simulink model "main"  (R2018b)
settings: Solver=VariableStepAuto  StartTime=0.0  StopTime=200  RelTol=1e-3
libraries: simulink x6, aerolibutil x2, sharedtransform x2
settings Model: SimulationMode=accelerator  Creator=exote  LastModifiedBy=exote

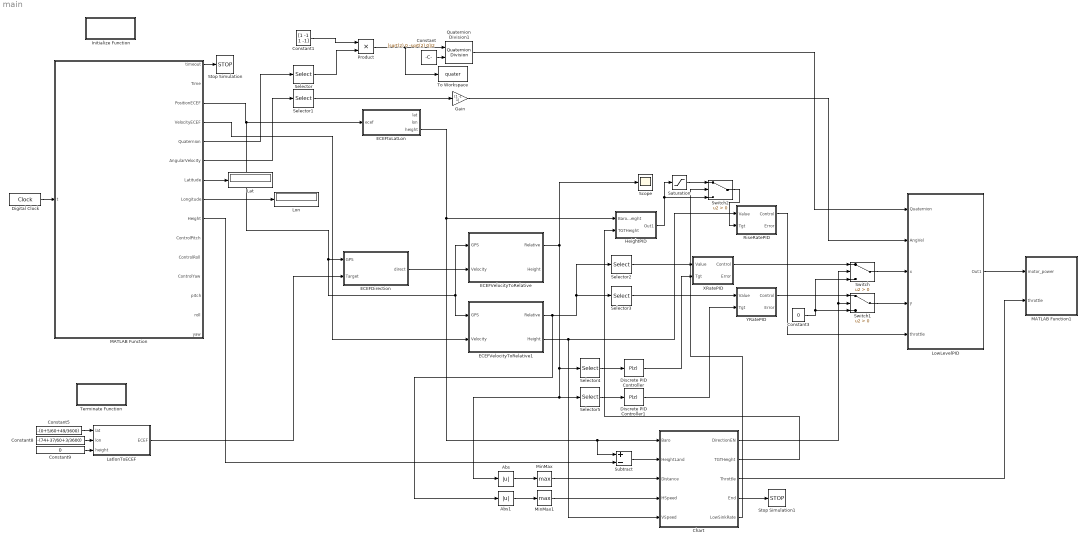
== system main ==
  Abs : Abs
  Abs1 : Abs
  Chart : Stateflow chart  TreatAsAtomicUnit=on
  Constant : Constant  Value=[sqrt(2) 0 -sqrt(2) 0]/2
  Constant1 : Constant  Value=[1 -1 1 -1]
  Constant3 : Constant  Value=0
  Constant5 : Constant  Value=-(0+5/60+49/3600)
  Constant8 : Constant  Value=-(74+37/60+3/3600)
  Constant9 : Constant  Value=0
  Digital Clock : DigitalClock  SampleTime=0.01
  Discrete PID Controller : simulink/Continuous/PID Controller  Controller=P  Form=Parallel  TimeDomain=Discrete-time  SampleTime=-1  IntegratorMethod=Forward Euler  FilterMethod=Forward Euler  ControllerParametersSource=internal  P=-0.1  I=0  D=0  UseFilter=on  N=100  TunerSelectOption=Transfer Function Based (PID Tuner App)  InitialConditionSource=internal  InitialConditionForIntegrator=0  InitialConditionForFilter=0  DifferentiatorICPrevScaledInput=0  ExternalReset=none  TrackingMode=off  Kt=1  LimitOutput=on  UpperSaturationLimit=20  LowerSaturationLimit=-20  LinearizeAsGain=off  AntiWindupMode=none  Kb=1  POutMin=[]  POutMax=[]  IOutMin=[]  IOutMax=[]  DOutMin=[]  DOutMax=[]  NOutMin=[]  NOutMax=[]  SumOutMin=[]  SumOutMax=[]  SaturationOutMin=[]  SaturationOutMax=[]  PParamMin=[]  PParamMax=[]  IParamMin=[]  IParamMax=[]  DParamMin=[]  DParamMax=[]  NParamMin=[]  NParamMax=[]  KbParamMin=[]  KbParamMax=[]  KtParamMin=[]  KtParamMax=[]  KbOutMin=[]  KbOutMax=[]  KtOutMin=[]  KtOutMax=[]  IntegratorOutMin=[]  IntegratorOutMax=[]  FilterOutMin=[]  FilterOutMax=[]  SumI1OutMin=[]  SumI1OutMax=[]  SumI2OutMin=[]  SumI2OutMax=[]  SumI3OutMin=[]  SumI3OutMax=[]  SumI4OutMin=[]  SumI4OutMax=[]  SumDOutMin=[]  SumDOutMax=[]  DifferentiatorOutMin=[]  DifferentiatorOutMax=[]  FilterDiffOutCoefMin=[]  FilterDiffOutCoefMax=[]  ReciprocalOutMin=[]  ReciprocalOutMax=[]  SumDenOutMin=[]  SumDenOutMax=[]  SumNumOutMin=[]  SumNumOutMax=[]  DivideOutMin=[]  DivideOutMax=[]  IntegratorContinuousStateAttributes=''  IntegratorStateMustResolveToSignalObject=off  IntegratorRTWStateStorageClass=Auto  FilterContinuousStateAttributes=''  FilterStateMustResolveToSignalObject=off  FilterRTWStateStorageClass=Auto  ParallelPVariant=InternalParameters  IdealPVariant=Disabled  IVariant=Disabled  DVariant=Disabled  IntegratorVariant=Disabled  SatVariant=Enabled  AWVariant=Disabled  PCopyVariant=Disabled  TRVariant=Disabled  FdbkBlocksVariant=Forward  IdealPFdbkVariant=Disabled  SatFdbkVariant=Disabled  DerivativeFilterVariant=Disabled  NVariant=Disabled  NCopyVariant=Disabled_SignalSpec  FilterICVariant=Disabled  IntegratorICVariant=Disabled  ExternalResetVariant=Disabled  TRSumVariant=Passthrough  SumFdbkVariant=Disabled  SumVariant=Passthrough_P
  Discrete PID Controller1 : simulink/Continuous/PID Controller  Controller=P  Form=Parallel  TimeDomain=Discrete-time  SampleTime=-1  IntegratorMethod=Forward Euler  FilterMethod=Forward Euler  ControllerParametersSource=internal  P=-0.1  I=0  D=0  UseFilter=on  N=100  TunerSelectOption=Transfer Function Based (PID Tuner App)  InitialConditionSource=internal  InitialConditionForIntegrator=0  InitialConditionForFilter=0  DifferentiatorICPrevScaledInput=0  ExternalReset=none  TrackingMode=off  Kt=1  LimitOutput=on  UpperSaturationLimit=20  LowerSaturationLimit=-20  LinearizeAsGain=off  AntiWindupMode=none  Kb=1  POutMin=[]  POutMax=[]  IOutMin=[]  IOutMax=[]  DOutMin=[]  DOutMax=[]  NOutMin=[]  NOutMax=[]  SumOutMin=[]  SumOutMax=[]  SaturationOutMin=[]  SaturationOutMax=[]  PParamMin=[]  PParamMax=[]  IParamMin=[]  IParamMax=[]  DParamMin=[]  DParamMax=[]  NParamMin=[]  NParamMax=[]  KbParamMin=[]  KbParamMax=[]  KtParamMin=[]  KtParamMax=[]  KbOutMin=[]  KbOutMax=[]  KtOutMin=[]  KtOutMax=[]  IntegratorOutMin=[]  IntegratorOutMax=[]  FilterOutMin=[]  FilterOutMax=[]  SumI1OutMin=[]  SumI1OutMax=[]  SumI2OutMin=[]  SumI2OutMax=[]  SumI3OutMin=[]  SumI3OutMax=[]  SumI4OutMin=[]  SumI4OutMax=[]  SumDOutMin=[]  SumDOutMax=[]  DifferentiatorOutMin=[]  DifferentiatorOutMax=[]  FilterDiffOutCoefMin=[]  FilterDiffOutCoefMax=[]  ReciprocalOutMin=[]  ReciprocalOutMax=[]  SumDenOutMin=[]  SumDenOutMax=[]  SumNumOutMin=[]  SumNumOutMax=[]  DivideOutMin=[]  DivideOutMax=[]  IntegratorContinuousStateAttributes=''  IntegratorStateMustResolveToSignalObject=off  IntegratorRTWStateStorageClass=Auto  FilterContinuousStateAttributes=''  FilterStateMustResolveToSignalObject=off  FilterRTWStateStorageClass=Auto  ParallelPVariant=InternalParameters  IdealPVariant=Disabled  IVariant=Disabled  DVariant=Disabled  IntegratorVariant=Disabled  SatVariant=Enabled  AWVariant=Disabled  PCopyVariant=Disabled  TRVariant=Disabled  FdbkBlocksVariant=Forward  IdealPFdbkVariant=Disabled  SatFdbkVariant=Disabled  DerivativeFilterVariant=Disabled  NVariant=Disabled  NCopyVariant=Disabled_SignalSpec  FilterICVariant=Disabled  IntegratorICVariant=Disabled  ExternalResetVariant=Disabled  TRSumVariant=Passthrough  SumFdbkVariant=Disabled  SumVariant=Passthrough_P
  ECEFDirection : MATLAB Function  TreatAsAtomicUnit=on
  ECEFVelocityToRelative : MATLAB Function  TreatAsAtomicUnit=on
  ECEFVelocityToRelative1 : MATLAB Function  TreatAsAtomicUnit=on
  ECEFtoLatLon : MATLAB Function  TreatAsAtomicUnit=on
  Gain : Gain  Gain=[1 -1 1]
  HeightPID : Subsystem
  Initialize Function : Subsystem  TreatAsAtomicUnit=on
  Lat : Display
  "LatlonToECEF " : MATLAB Function  TreatAsAtomicUnit=on
  Lon : Display
  "LowLevelPID " : Subsystem
  MATLAB Function : MATLAB Function  TreatAsAtomicUnit=on
  MATLAB Function1 : MATLAB Function  TreatAsAtomicUnit=on
  MinMax : MinMax  Function=max
  MinMax1 : MinMax  Function=max
  Product : Product
  Quaternion Division1 : aerolibutil/Quaternion Division
      settings: SourceProductName=Aerospace Blockset  SourceProductBaseCode=AE
  "RiseRatePID " : Subsystem
  Saturation : Saturate  UpperLimit=inf
  Scope : Scope
  Selector : Selector  InputPortWidth=4  IndexOptions=Index vector (dialog)  Indices=[4 1 2 3]  OutputSizes=1
  Selector1 : Selector  InputPortWidth=3  IndexOptions=Index vector (dialog)  Indices=[1 3 2]  OutputSizes=1
  Selector2 : Selector  InputPortWidth=2  IndexOptions=Index vector (dialog)  Indices=1  OutputSizes=1
  Selector3 : Selector  InputPortWidth=2  IndexOptions=Index vector (dialog)  Indices=2  OutputSizes=1
  Selector4 : Selector  InputPortWidth=2  IndexOptions=Index vector (dialog)  Indices=1  OutputSizes=1
  Selector5 : Selector  InputPortWidth=2  IndexOptions=Index vector (dialog)  Indices=2  OutputSizes=1
  Stop Simulation : Stop
  Stop Simulation1 : Stop
  Subtract : Sum  Inputs=+-
  Switch : Switch  Criteria=u2 > Threshold
  Switch1 : Switch  Criteria=u2 > Threshold
  Switch2 : Switch  Criteria=u2 > Threshold
  Terminate Function : Subsystem  TreatAsAtomicUnit=on
  To Workspace : ToWorkspace  VariableName=quater  SampleTime=-1
      settings: Save2DSignal=2-D array (concatenate along first dimension)
  XRatePID : Subsystem
  YRatePID : Subsystem
  wires:
  Digital Clock/1 -> MATLAB Function/1(t)
  MATLAB Function/1(timeout) -> Stop Simulation/1
  Selector/1 -> Product/2
  Constant/1 -> Quaternion Division1/2
  MATLAB Function/5(Quaternion) -> Selector/1
  MATLAB Function/6(AngularVelocity) -> Selector1/1
  Constant1/1 -> Product/1
  Product/1 -> Quaternion Division1/1, To Workspace/1
  Quaternion Division1/1 -> "LowLevelPID "/1("Quaternion ")
  "LowLevelPID "/1(Out1) -> MATLAB Function1/1(motor_power)
  MATLAB Function/7(Latitude) -> Lat/1
  MATLAB Function/8(Longitude) -> Lon/1
  Gain/1 -> "LowLevelPID "/2(AngVel)
  Selector1/1 -> Gain/1
  MATLAB Function/3(PositionECEF) -> ECEFtoLatLon/1(ecef), ECEFVelocityToRelative/1(GPS), ECEFVelocityToRelative1/1(GPS), ECEFDirection/1(GPS)
  MATLAB Function/4(VelocityECEF) -> ECEFVelocityToRelative1/2(Velocity)
  "RiseRatePID "/1(Control) -> "LowLevelPID "/5(throttle)
  ECEFtoLatLon/3(height) -> Chart/1(Baro), Subtract/1, HeightPID/1(BaroHeight)
  Chart/2(TGTHeight) -> HeightPID/2(TGTHeight)
  Constant5/1 -> "LatlonToECEF "/1(lat)
  Constant8/1 -> "LatlonToECEF "/2(lon)
  Constant9/1 -> "LatlonToECEF "/3(height)
  "LatlonToECEF "/1(ECEF) -> ECEFDirection/2(Target)
  ECEFDirection/1(direct) -> ECEFVelocityToRelative/2(Velocity)
  ECEFVelocityToRelative1/2(Height) -> "RiseRatePID "/1("Value "), Chart/5(VSpeed)
  Selector2/1 -> XRatePID/1("Value ")
  Selector3/1 -> YRatePID/1("Value ")
  ECEFVelocityToRelative1/1(Relative) -> Abs1/1, Selector3/1, Selector2/1
  HeightPID/1(Out1) -> Switch2/3, Saturation/1
  YRatePID/1(Control) -> Switch1/1
  XRatePID/1(Control) -> Switch/1
  Selector4/1 -> Discrete PID Controller/1
  Selector5/1 -> Discrete PID Controller1/1
  ECEFVelocityToRelative/1(Relative) -> Abs/1, Selector5/1, Selector4/1, Scope/1
  Discrete PID Controller/1 -> XRatePID/2(Tgt)
  Discrete PID Controller1/1 -> YRatePID/2(Tgt)
  Switch1/1 -> "LowLevelPID "/4(y)
  Switch/1 -> "LowLevelPID "/3(x)
  Constant3/1 -> Switch1/3, Switch/3
  Chart/1(DirectionEN) -> Switch1/2, Switch/2
  Chart/3(Throttle) -> MATLAB Function1/2(throttle)
  MATLAB Function/9(Height) -> Subtract/2
  MinMax/1 -> Chart/3(Distance)
  MinMax1/1 -> Chart/4(HSpeed)
  Chart/4(End) -> Stop Simulation1/1
  Subtract/1 -> Chart/2(HeightLand)
  Abs/1 -> MinMax/1
  Abs1/1 -> MinMax1/1
  Switch2/1 -> "RiseRatePID "/2(Tgt)
  Saturation/1 -> Switch2/1
  Chart/5(LowSinkRate) -> Switch2/2

== system main/HeightPID ==
  BaroHeight : Inport
  TGTHeight : Inport  Port=2
  Discrete PID Controller : simulink/Continuous/PID Controller  Controller=PI  Form=Parallel  TimeDomain=Discrete-time  SampleTime=-1  IntegratorMethod=Forward Euler  FilterMethod=Forward Euler  ControllerParametersSource=internal  P=0.5  I=0  D=0  UseFilter=off  N=100  TunerSelectOption=Transfer Function Based (PID Tuner App)  InitialConditionSource=internal  InitialConditionForIntegrator=0  InitialConditionForFilter=0  DifferentiatorICPrevScaledInput=0  ExternalReset=none  TrackingMode=off  Kt=1  LimitOutput=on  UpperSaturationLimit=20  LowerSaturationLimit=-20  LinearizeAsGain=off  AntiWindupMode=none  Kb=1  POutMin=[]  POutMax=[]  IOutMin=[]  IOutMax=[]  DOutMin=[]  DOutMax=[]  NOutMin=[]  NOutMax=[]  SumOutMin=[]  SumOutMax=[]  SaturationOutMin=[]  SaturationOutMax=[]  PParamMin=[]  PParamMax=[]  IParamMin=[]  IParamMax=[]  DParamMin=[]  DParamMax=[]  NParamMin=[]  NParamMax=[]  KbParamMin=[]  KbParamMax=[]  KtParamMin=[]  KtParamMax=[]  KbOutMin=[]  KbOutMax=[]  KtOutMin=[]  KtOutMax=[]  IntegratorOutMin=[]  IntegratorOutMax=[]  FilterOutMin=[]  FilterOutMax=[]  SumI1OutMin=[]  SumI1OutMax=[]  SumI2OutMin=[]  SumI2OutMax=[]  SumI3OutMin=[]  SumI3OutMax=[]  SumI4OutMin=[]  SumI4OutMax=[]  SumDOutMin=[]  SumDOutMax=[]  DifferentiatorOutMin=[]  DifferentiatorOutMax=[]  FilterDiffOutCoefMin=[]  FilterDiffOutCoefMax=[]  ReciprocalOutMin=[]  ReciprocalOutMax=[]  SumDenOutMin=[]  SumDenOutMax=[]  SumNumOutMin=[]  SumNumOutMax=[]  DivideOutMin=[]  DivideOutMax=[]  IntegratorContinuousStateAttributes=''  IntegratorStateMustResolveToSignalObject=off  IntegratorRTWStateStorageClass=Auto  FilterContinuousStateAttributes=''  FilterStateMustResolveToSignalObject=off  FilterRTWStateStorageClass=Auto  ParallelPVariant=InternalParameters  IdealPVariant=Disabled  IVariant=InternalParameters  DVariant=Disabled  IntegratorVariant=Discrete  SatVariant=Enabled  AWVariant=Passthrough  PCopyVariant=Disabled  TRVariant=Disabled  FdbkBlocksVariant=Forward  IdealPFdbkVariant=Disabled  SatFdbkVariant=Disabled  DerivativeFilterVariant=Disabled  NVariant=Disabled  NCopyVariant=Disabled_SignalSpec  FilterICVariant=Disabled  IntegratorICVariant=InternalICs  ExternalResetVariant=Disabled  TRSumVariant=Passthrough  SumFdbkVariant=Disabled  SumVariant=Sum_PI
  Subtract2 : Sum  Inputs=+-
  Out1 : Outport
  wires:
  Subtract2/1 -> Discrete PID Controller/1
  BaroHeight/1 -> Subtract2/2
  Discrete PID Controller/1 -> Out1/1
  TGTHeight/1 -> Subtract2/1

== system main/Initialize Function ==
  Event Listener : EventListener  DisableCoverage=on  EventName=reset
  MATLAB Function : MATLAB Function  TreatAsAtomicUnit=on

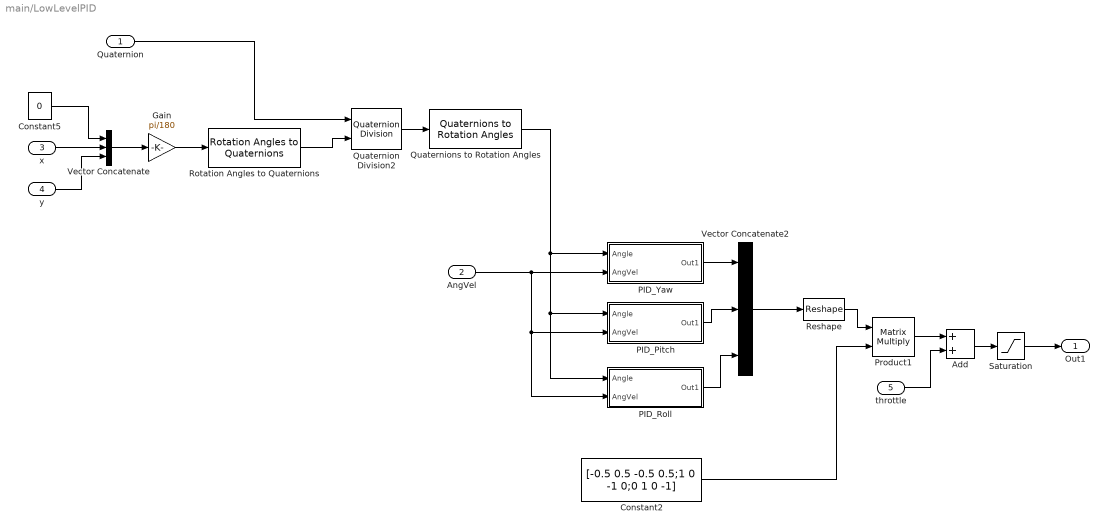
== system main/LowLevelPID  ==
  "Quaternion " : Inport
  AngVel : Inport  Port=2
  x : Inport  Port=3
  y : Inport  Port=4
  throttle : Inport  Port=5
  Add : Sum
  Constant2 : Constant  Value=[-0.5 0.5 -0.5 0.5;1 0 -1 0;0 1 0 -1]
  Constant5 : Constant  Value=0
  Gain : Gain  Gain=pi/180
  PID_Pitch : Subsystem
  PID_Roll : Subsystem
  PID_Yaw : Subsystem
  Product1 : Product  Multiplication=Matrix(*)
  Quaternion Division2 : aerolibutil/Quaternion Division
      settings: SourceProductName=Aerospace Blockset  SourceProductBaseCode=AE
  Quaternions to Rotation Angles : sharedtransform/Quaternions to Rotation Angles  rotationOrder=ZXY  aMode=aMode
      settings: SourceProductBaseCode=AE
  Reshape : Reshape  OutputDimensionality=Customize  OutputDimensions=[1,3]
  Rotation Angles to Quaternions : sharedtransform/Rotation Angles to Quaternions  rotationOrder=ZXY  aMode=aMode
      settings: SourceProductName=Aerospace Blockset  SourceProductBaseCode=AE
  Saturation : Saturate  UpperLimit=1  LowerLimit=0
  Vector Concatenate : Concatenate  NumInputs=3
  Vector Concatenate2 : Concatenate  NumInputs=3
  Out1 : Outport
  wires:
  Product1/1 -> Add/1
  Quaternions to Rotation Angles/1 -> PID_Pitch/1(Angle), PID_Roll/1(Angle), PID_Yaw/1(Angle)
  Vector Concatenate2/1 -> Reshape/1
  Constant2/1 -> Product1/2
  Reshape/1 -> Product1/1
  Add/1 -> Saturation/1
  "Quaternion "/1 -> Quaternion Division2/1
  Rotation Angles to Quaternions/1 -> Quaternion Division2/2
  Quaternion Division2/1 -> Quaternions to Rotation Angles/1
  Saturation/1 -> Out1/1
  throttle/1 -> Add/2
  Vector Concatenate/1 -> Gain/1
  x/1 -> Vector Concatenate/2
  y/1 -> Vector Concatenate/3
  Constant5/1 -> Vector Concatenate/1
  Gain/1 -> Rotation Angles to Quaternions/1
  AngVel/1 -> PID_Roll/2(AngVel), PID_Pitch/2(AngVel), PID_Yaw/2(AngVel)
  PID_Yaw/1(Out1) -> Vector Concatenate2/1
  PID_Pitch/1(Out1) -> Vector Concatenate2/2
  PID_Roll/1(Out1) -> Vector Concatenate2/3

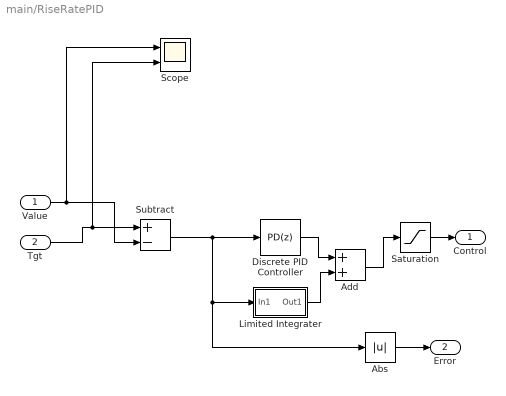
== system main/RiseRatePID  ==
  "Value " : Inport
  Tgt : Inport  Port=2
  Abs : Abs
  Add : Sum
  Discrete PID Controller : simulink/Continuous/PID Controller  Controller=PD  Form=Parallel  TimeDomain=Discrete-time  SampleTime=-1  IntegratorMethod=Forward Euler  FilterMethod=Forward Euler  ControllerParametersSource=internal  P=1  I=1  D=0.01  UseFilter=on  N=30  TunerSelectOption=Transfer Function Based (PID Tuner App)  InitialConditionSource=internal  InitialConditionForIntegrator=0  InitialConditionForFilter=0  DifferentiatorICPrevScaledInput=0  ExternalReset=none  TrackingMode=off  Kt=1  LimitOutput=off  UpperSaturationLimit=0.75  LowerSaturationLimit=0.25  LinearizeAsGain=off  AntiWindupMode=none  Kb=1  POutMin=[]  POutMax=[]  IOutMin=[-100]  IOutMax=[100]  DOutMin=[]  DOutMax=[]  NOutMin=[]  NOutMax=[]  SumOutMin=[]  SumOutMax=[]  SaturationOutMin=[]  SaturationOutMax=[]  PParamMin=[]  PParamMax=[]  IParamMin=[]  IParamMax=[]  DParamMin=[]  DParamMax=[]  NParamMin=[]  NParamMax=[]  KbParamMin=[]  KbParamMax=[]  KtParamMin=[]  KtParamMax=[]  KbOutMin=[]  KbOutMax=[]  KtOutMin=[]  KtOutMax=[]  IntegratorOutMin=[]  IntegratorOutMax=[]  FilterOutMin=[]  FilterOutMax=[]  SumI1OutMin=[]  SumI1OutMax=[]  SumI2OutMin=[]  SumI2OutMax=[]  SumI3OutMin=[]  SumI3OutMax=[]  SumI4OutMin=[]  SumI4OutMax=[]  SumDOutMin=[]  SumDOutMax=[]  DifferentiatorOutMin=[]  DifferentiatorOutMax=[]  FilterDiffOutCoefMin=[]  FilterDiffOutCoefMax=[]  ReciprocalOutMin=[]  ReciprocalOutMax=[]  SumDenOutMin=[]  SumDenOutMax=[]  SumNumOutMin=[]  SumNumOutMax=[]  DivideOutMin=[]  DivideOutMax=[]  IntegratorContinuousStateAttributes=''  IntegratorStateMustResolveToSignalObject=off  IntegratorRTWStateStorageClass=Auto  FilterContinuousStateAttributes=''  FilterStateMustResolveToSignalObject=off  FilterRTWStateStorageClass=Auto  ParallelPVariant=InternalParameters  IdealPVariant=Disabled  IVariant=Disabled  DVariant=InternalParameters  IntegratorVariant=Disabled  SatVariant=Disabled  AWVariant=Disabled  PCopyVariant=Disabled  TRVariant=Disabled  FdbkBlocksVariant=Forward  IdealPFdbkVariant=Disabled  SatFdbkVariant=Disabled  DerivativeFilterVariant=ForwardEulerFilter  NVariant=InternalParameters  NCopyVariant=Disabled  FilterICVariant=InternalICsFilter  IntegratorICVariant=Disabled  ExternalResetVariant=Disabled  TRSumVariant=Passthrough  SumFdbkVariant=Disabled  SumVariant=Sum_PD
  Limited Integrater : Subsystem
  Saturation : Saturate  UpperLimit=0.75  LowerLimit=0.25
  Scope : Scope  NumInputPorts=2
  Subtract : Sum  Inputs=+-
  Control : Outport
  Error : Outport  Port=2
  wires:
  Subtract/1 -> Discrete PID Controller/1, Abs/1, Limited Integrater/1(In1)
  Tgt/1 -> Scope/2, Subtract/1
  Saturation/1 -> Control/1
  Discrete PID Controller/1 -> Add/1
  Limited Integrater/1(Out1) -> Add/2
  Add/1 -> Saturation/1
  "Value "/1 -> Scope/1, Subtract/2
  Abs/1 -> Error/1

== system main/Terminate Function ==
  Event Listener : EventListener  DisableCoverage=on  EventType=Terminate  EventName=reset
  MATLAB Function : MATLAB Function  TreatAsAtomicUnit=on

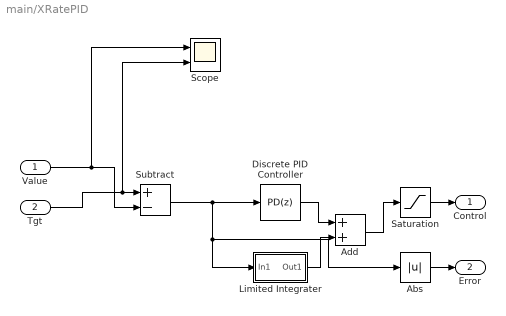
== system main/XRatePID ==
  "Value " : Inport
  Tgt : Inport  Port=2
  Abs : Abs
  Add : Sum
  Discrete PID Controller : simulink/Continuous/PID Controller  Controller=PD  Form=Parallel  TimeDomain=Discrete-time  SampleTime=-1  IntegratorMethod=Forward Euler  FilterMethod=Forward Euler  ControllerParametersSource=internal  P=-5  I=1  D=0  UseFilter=on  N=30  TunerSelectOption=Transfer Function Based (PID Tuner App)  InitialConditionSource=internal  InitialConditionForIntegrator=0  InitialConditionForFilter=0  DifferentiatorICPrevScaledInput=0  ExternalReset=none  TrackingMode=off  Kt=1  LimitOutput=off  UpperSaturationLimit=0.75  LowerSaturationLimit=0.25  LinearizeAsGain=off  AntiWindupMode=none  Kb=1  POutMin=[]  POutMax=[]  IOutMin=[-100]  IOutMax=[100]  DOutMin=[]  DOutMax=[]  NOutMin=[]  NOutMax=[]  SumOutMin=[]  SumOutMax=[]  SaturationOutMin=[]  SaturationOutMax=[]  PParamMin=[]  PParamMax=[]  IParamMin=[]  IParamMax=[]  DParamMin=[]  DParamMax=[]  NParamMin=[]  NParamMax=[]  KbParamMin=[]  KbParamMax=[]  KtParamMin=[]  KtParamMax=[]  KbOutMin=[]  KbOutMax=[]  KtOutMin=[]  KtOutMax=[]  IntegratorOutMin=[]  IntegratorOutMax=[]  FilterOutMin=[]  FilterOutMax=[]  SumI1OutMin=[]  SumI1OutMax=[]  SumI2OutMin=[]  SumI2OutMax=[]  SumI3OutMin=[]  SumI3OutMax=[]  SumI4OutMin=[]  SumI4OutMax=[]  SumDOutMin=[]  SumDOutMax=[]  DifferentiatorOutMin=[]  DifferentiatorOutMax=[]  FilterDiffOutCoefMin=[]  FilterDiffOutCoefMax=[]  ReciprocalOutMin=[]  ReciprocalOutMax=[]  SumDenOutMin=[]  SumDenOutMax=[]  SumNumOutMin=[]  SumNumOutMax=[]  DivideOutMin=[]  DivideOutMax=[]  IntegratorContinuousStateAttributes=''  IntegratorStateMustResolveToSignalObject=off  IntegratorRTWStateStorageClass=Auto  FilterContinuousStateAttributes=''  FilterStateMustResolveToSignalObject=off  FilterRTWStateStorageClass=Auto  ParallelPVariant=InternalParameters  IdealPVariant=Disabled  IVariant=Disabled  DVariant=InternalParameters  IntegratorVariant=Disabled  SatVariant=Disabled  AWVariant=Disabled  PCopyVariant=Disabled  TRVariant=Disabled  FdbkBlocksVariant=Forward  IdealPFdbkVariant=Disabled  SatFdbkVariant=Disabled  DerivativeFilterVariant=ForwardEulerFilter  NVariant=InternalParameters  NCopyVariant=Disabled  FilterICVariant=InternalICsFilter  IntegratorICVariant=Disabled  ExternalResetVariant=Disabled  TRSumVariant=Passthrough  SumFdbkVariant=Disabled  SumVariant=Sum_PD
  Limited Integrater : Subsystem
  Saturation : Saturate  UpperLimit=10  LowerLimit=-10
  Scope : Scope  NumInputPorts=2
  Subtract : Sum  Inputs=+-
  Control : Outport
  Error : Outport  Port=2
  wires:
  Subtract/1 -> Discrete PID Controller/1, Abs/1, Limited Integrater/1(In1)
  Tgt/1 -> Scope/2, Subtract/1
  Saturation/1 -> Control/1
  Discrete PID Controller/1 -> Add/1
  Limited Integrater/1(Out1) -> Add/2
  Add/1 -> Saturation/1
  "Value "/1 -> Scope/1, Subtract/2
  Abs/1 -> Error/1

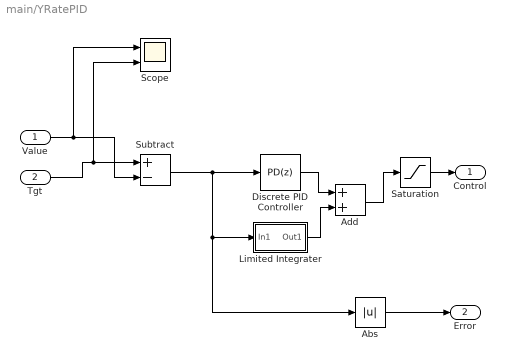
== system main/YRatePID ==
  "Value " : Inport
  Tgt : Inport  Port=2
  Abs : Abs
  Add : Sum
  Discrete PID Controller : simulink/Continuous/PID Controller  Controller=PD  Form=Parallel  TimeDomain=Discrete-time  SampleTime=-1  IntegratorMethod=Forward Euler  FilterMethod=Forward Euler  ControllerParametersSource=internal  P=-5  I=1  D=0  UseFilter=on  N=30  TunerSelectOption=Transfer Function Based (PID Tuner App)  InitialConditionSource=internal  InitialConditionForIntegrator=0  InitialConditionForFilter=0  DifferentiatorICPrevScaledInput=0  ExternalReset=none  TrackingMode=off  Kt=1  LimitOutput=off  UpperSaturationLimit=0.75  LowerSaturationLimit=0.25  LinearizeAsGain=off  AntiWindupMode=none  Kb=1  POutMin=[]  POutMax=[]  IOutMin=[-100]  IOutMax=[100]  DOutMin=[]  DOutMax=[]  NOutMin=[]  NOutMax=[]  SumOutMin=[]  SumOutMax=[]  SaturationOutMin=[]  SaturationOutMax=[]  PParamMin=[]  PParamMax=[]  IParamMin=[]  IParamMax=[]  DParamMin=[]  DParamMax=[]  NParamMin=[]  NParamMax=[]  KbParamMin=[]  KbParamMax=[]  KtParamMin=[]  KtParamMax=[]  KbOutMin=[]  KbOutMax=[]  KtOutMin=[]  KtOutMax=[]  IntegratorOutMin=[]  IntegratorOutMax=[]  FilterOutMin=[]  FilterOutMax=[]  SumI1OutMin=[]  SumI1OutMax=[]  SumI2OutMin=[]  SumI2OutMax=[]  SumI3OutMin=[]  SumI3OutMax=[]  SumI4OutMin=[]  SumI4OutMax=[]  SumDOutMin=[]  SumDOutMax=[]  DifferentiatorOutMin=[]  DifferentiatorOutMax=[]  FilterDiffOutCoefMin=[]  FilterDiffOutCoefMax=[]  ReciprocalOutMin=[]  ReciprocalOutMax=[]  SumDenOutMin=[]  SumDenOutMax=[]  SumNumOutMin=[]  SumNumOutMax=[]  DivideOutMin=[]  DivideOutMax=[]  IntegratorContinuousStateAttributes=''  IntegratorStateMustResolveToSignalObject=off  IntegratorRTWStateStorageClass=Auto  FilterContinuousStateAttributes=''  FilterStateMustResolveToSignalObject=off  FilterRTWStateStorageClass=Auto  ParallelPVariant=InternalParameters  IdealPVariant=Disabled  IVariant=Disabled  DVariant=InternalParameters  IntegratorVariant=Disabled  SatVariant=Disabled  AWVariant=Disabled  PCopyVariant=Disabled  TRVariant=Disabled  FdbkBlocksVariant=Forward  IdealPFdbkVariant=Disabled  SatFdbkVariant=Disabled  DerivativeFilterVariant=ForwardEulerFilter  NVariant=InternalParameters  NCopyVariant=Disabled  FilterICVariant=InternalICsFilter  IntegratorICVariant=Disabled  ExternalResetVariant=Disabled  TRSumVariant=Passthrough  SumFdbkVariant=Disabled  SumVariant=Sum_PD
  Limited Integrater : Subsystem
  Saturation : Saturate  UpperLimit=10  LowerLimit=-10
  Scope : Scope  NumInputPorts=2
  Subtract : Sum  Inputs=+-
  Control : Outport
  Error : Outport  Port=2
  wires:
  Subtract/1 -> Discrete PID Controller/1, Abs/1, Limited Integrater/1(In1)
  Tgt/1 -> Scope/2, Subtract/1
  Saturation/1 -> Control/1
  Discrete PID Controller/1 -> Add/1
  Limited Integrater/1(Out1) -> Add/2
  Add/1 -> Saturation/1
  "Value "/1 -> Scope/1, Subtract/2
  Abs/1 -> Error/1

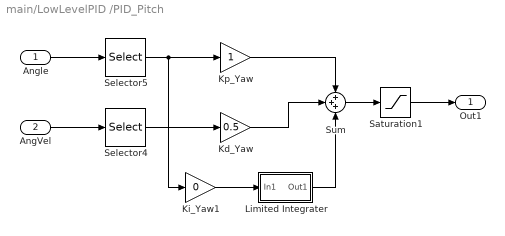
== system main/LowLevelPID /PID_Pitch ==
  Angle : Inport
  AngVel : Inport  Port=2
  Kd_Yaw : Gain  Gain=0.5
  Ki_Yaw1 : Gain  Gain=0
  Kp_Yaw : Gain
  Limited Integrater : Subsystem
  Saturation1 : Saturate
  Selector4 : Selector  InputPortWidth=3  IndexOptions=Index vector (dialog)  Indices=2  OutputSizes=1
  Selector5 : Selector  InputPortWidth=3  IndexOptions=Index vector (dialog)  Indices=2  OutputSizes=1
  Sum : Sum  Inputs=+++
  Out1 : Outport
  wires:
  Ki_Yaw1/1 -> Limited Integrater/1(In1)
  Limited Integrater/1(Out1) -> Sum/3
  Angle/1 -> Selector5/1
  Sum/1 -> Saturation1/1
  Kd_Yaw/1 -> Sum/2
  Selector5/1 -> Ki_Yaw1/1, Kp_Yaw/1
  Kp_Yaw/1 -> Sum/1
  Selector4/1 -> Kd_Yaw/1
  AngVel/1 -> Selector4/1
  Saturation1/1 -> Out1/1

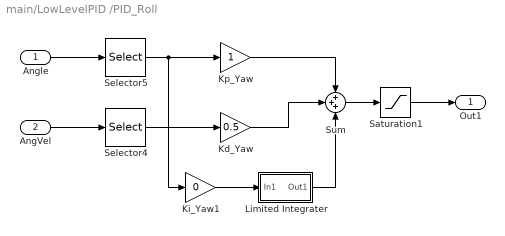
== system main/LowLevelPID /PID_Roll ==
  Angle : Inport
  AngVel : Inport  Port=2
  Kd_Yaw : Gain  Gain=0.5
  Ki_Yaw1 : Gain  Gain=0
  Kp_Yaw : Gain
  Limited Integrater : Subsystem
  Saturation1 : Saturate
  Selector4 : Selector  InputPortWidth=3  IndexOptions=Index vector (dialog)  Indices=3  OutputSizes=1
  Selector5 : Selector  InputPortWidth=3  IndexOptions=Index vector (dialog)  Indices=3  OutputSizes=1
  Sum : Sum  Inputs=+++
  Out1 : Outport
  wires:
  Ki_Yaw1/1 -> Limited Integrater/1(In1)
  Limited Integrater/1(Out1) -> Sum/3
  Angle/1 -> Selector5/1
  Sum/1 -> Saturation1/1
  Kd_Yaw/1 -> Sum/2
  Selector5/1 -> Ki_Yaw1/1, Kp_Yaw/1
  Kp_Yaw/1 -> Sum/1
  Selector4/1 -> Kd_Yaw/1
  AngVel/1 -> Selector4/1
  Saturation1/1 -> Out1/1

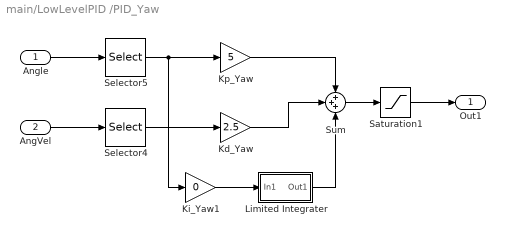
== system main/LowLevelPID /PID_Yaw ==
  Angle : Inport
  AngVel : Inport  Port=2
  Kd_Yaw : Gain  Gain=2.5
  Ki_Yaw1 : Gain  Gain=0
  Kp_Yaw : Gain  Gain=5
  Limited Integrater : Subsystem
  Saturation1 : Saturate
  Selector4 : Selector  InputPortWidth=3  IndexOptions=Index vector (dialog)  Indices=1  OutputSizes=1
  Selector5 : Selector  InputPortWidth=3  IndexOptions=Index vector (dialog)  Indices=1  OutputSizes=1
  Sum : Sum  Inputs=+++
  Out1 : Outport
  wires:
  Ki_Yaw1/1 -> Limited Integrater/1(In1)
  Limited Integrater/1(Out1) -> Sum/3
  Angle/1 -> Selector5/1
  Sum/1 -> Saturation1/1
  Kd_Yaw/1 -> Sum/2
  Selector5/1 -> Ki_Yaw1/1, Kp_Yaw/1
  Kp_Yaw/1 -> Sum/1
  Selector4/1 -> Kd_Yaw/1
  AngVel/1 -> Selector4/1
  Saturation1/1 -> Out1/1

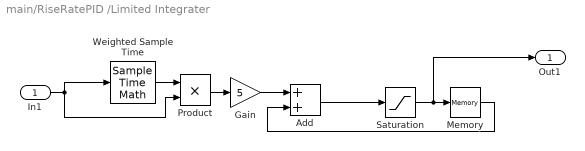
== system main/RiseRatePID /Limited Integrater ==
  In1 : Inport
  Add : Sum
  Gain : Gain  Gain=5
  Memory : Memory
  Product : Product
  Saturation : Saturate
  Weighted Sample Time : SampleTimeMath  TsampMathOp=Ts Only
  Out1 : Outport
  wires:
  Saturation/1 -> Out1/1, Memory/1
  Add/1 -> Saturation/1
  Memory/1 -> Add/2
  In1/1 -> Product/2, Weighted Sample Time/1
  Weighted Sample Time/1 -> Product/1
  Product/1 -> Gain/1
  Gain/1 -> Add/1

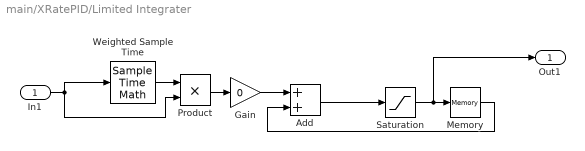
== system main/XRatePID/Limited Integrater ==
  In1 : Inport
  Add : Sum
  Gain : Gain  Gain=0
  Memory : Memory
  Product : Product
  Saturation : Saturate
  Weighted Sample Time : SampleTimeMath  TsampMathOp=Ts Only
  Out1 : Outport
  wires:
  Saturation/1 -> Out1/1, Memory/1
  Add/1 -> Saturation/1
  Memory/1 -> Add/2
  In1/1 -> Product/2, Weighted Sample Time/1
  Weighted Sample Time/1 -> Product/1
  Product/1 -> Gain/1
  Gain/1 -> Add/1

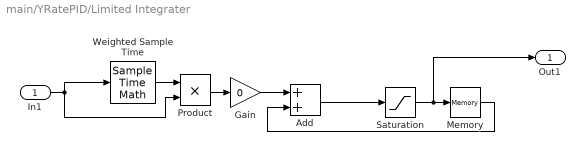
== system main/YRatePID/Limited Integrater ==
  In1 : Inport
  Add : Sum
  Gain : Gain  Gain=0
  Memory : Memory
  Product : Product
  Saturation : Saturate
  Weighted Sample Time : SampleTimeMath  TsampMathOp=Ts Only
  Out1 : Outport
  wires:
  Saturation/1 -> Out1/1, Memory/1
  Add/1 -> Saturation/1
  Memory/1 -> Add/2
  In1/1 -> Product/2, Weighted Sample Time/1
  Weighted Sample Time/1 -> Product/1
  Product/1 -> Gain/1
  Gain/1 -> Add/1

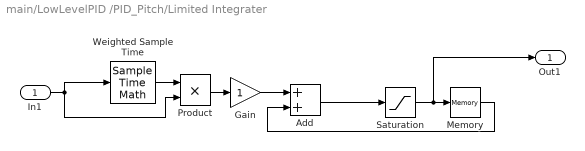
== system main/LowLevelPID /PID_Pitch/Limited Integrater ==
  In1 : Inport
  Add : Sum
  Gain : Gain
  Memory : Memory
  Product : Product
  Saturation : Saturate
  Weighted Sample Time : SampleTimeMath  TsampMathOp=Ts Only
  Out1 : Outport
  wires:
  Saturation/1 -> Out1/1, Memory/1
  Add/1 -> Saturation/1
  Memory/1 -> Add/2
  In1/1 -> Product/2, Weighted Sample Time/1
  Weighted Sample Time/1 -> Product/1
  Product/1 -> Gain/1
  Gain/1 -> Add/1

== system main/LowLevelPID /PID_Roll/Limited Integrater ==
  In1 : Inport
  Add : Sum
  Gain : Gain
  Memory : Memory
  Product : Product
  Saturation : Saturate
  Weighted Sample Time : SampleTimeMath  TsampMathOp=Ts Only
  Out1 : Outport
  wires:
  Saturation/1 -> Out1/1, Memory/1
  Add/1 -> Saturation/1
  Memory/1 -> Add/2
  In1/1 -> Product/2, Weighted Sample Time/1
  Weighted Sample Time/1 -> Product/1
  Product/1 -> Gain/1
  Gain/1 -> Add/1

== system main/LowLevelPID /PID_Yaw/Limited Integrater ==
  In1 : Inport
  Add : Sum
  Gain : Gain
  Memory : Memory
  Product : Product
  Saturation : Saturate
  Weighted Sample Time : SampleTimeMath  TsampMathOp=Ts Only
  Out1 : Outport
  wires:
  Saturation/1 -> Out1/1, Memory/1
  Add/1 -> Saturation/1
  Memory/1 -> Add/2
  In1/1 -> Product/2, Weighted Sample Time/1
  Weighted Sample Time/1 -> Product/1
  Product/1 -> Gain/1
  Gain/1 -> Add/1

== matlab function main/Initialize Function/MATLAB Function ==
function  KRPC_Init()
coder.extrinsic ('KRPC_Wrapper_Init');
KRPC_Wrapper_Init();

== matlab function main/MATLAB Function ==
  settings: updateMethod=DISCRETE
  data: timeout output size=1; Time output; PositionECEF output; VelocityECEF output; Quaternion output; AngularVelocity output; Latitude output; Longitude output; Height output; ControlPitch output; ControlRoll output; ControlYaw output; t input size=1; pitch output; roll output; yaw output
function [timeout,Time,PositionECEF,VelocityECEF,Quaternion,AngularVelocity, ...
    Latitude,Longitude,Height,ControlPitch,ControlRoll,ControlYaw ...
     ,pitch,roll,yaw]  = KRPC_GetData(t)

timeout = false;
Time = 0;
PositionECEF = zeros(1,3);
VelocityECEF = zeros(1,3);
Quaternion = zeros(1,4);
AngularVelocity = zeros(1,3);
Latitude=0;Longitude=0;Height=0;ControlPitch=0;ControlRoll=0;ControlYaw=0;
pitch = 0;roll=0;yaw=0;
coder.extrinsic ('KRPC_Wrapper_GetData');
[timeout,Time,PositionECEF,VelocityECEF,Quaternion,AngularVelocity, ...
    Latitude,Longitude,Height,ControlPitch,ControlRoll,ControlYaw ...
    ,pitch,roll,yaw]  = KRPC_Wrapper_GetData(t);
end

== matlab function main/Terminate Function/MATLAB Function ==
function  KRPC_DeInit()
coder.extrinsic ('KRPC_Wrapper_DeInit');
KRPC_Wrapper_DeInit();

== matlab function main/MATLAB Function1 ==
  data: motor_power input; throttle input
function KRPC_SetData(motor_power,throttle)
coder.extrinsic ('KRPC_Wrapper_SetData');
KRPC_Wrapper_SetData(motor_power,throttle);
end

== matlab function main/LatlonToECEF  ==
  data: lat input; ECEF output; lon input; height input
function ECEF = LatLontoECEF(lat,lon,height)
% lon(i) = atan2(ecef(i,2),ecef(i,1)) *180/pi;
% lat(i) = asin(ecef(i,2)/norm(ecef(i,:),2)) *180/pi;
ECEF = zeros(3,1);
ECEF(2) = sin(lat*pi/180)*(600e3+height);
r = cos(lat*pi/180)*(600e3+height);
ECEF(3) = sin(lon*pi/180) * r;
ECEF(1) = cos(lon*pi/180) * r;

== matlab function main/ECEFtoLatLon ==
  data: ecef input; lat output; lon output; height output
function [lat,lon,height] = ECEFtoLatLon(ecef)
lon = atan2(ecef(3),ecef(1)) *180/pi;
lat = asin(ecef(2)/norm(ecef,2)) *180/pi;
height = norm(ecef,2) - 600e3;

== matlab function main/ECEFDirection ==
  data: GPS input; direct output; Target input
function direct = ECEFDirection(GPS,Target)

GPS = reshape(GPS,1,[]);
Target = reshape(Target,1,[]);
% 统一高度
%GPS = 600e3 * GPS / norm(GPS);
%Target = 600e3 * Target / norm(Target);
% 过两点做弧
% 求角距离
sin_angdist = cross(GPS,Target) / (norm(GPS) * norm(Target));
dist = asin(norm(sin_angdist)) * 600e3;
%求方向向量
direct = cross(GPS,sin_angdist);
direct = direct/norm(direct);
direct = direct * dist;

== matlab function main/ECEFVelocityToRelative ==
  data: GPS input; Relative output; Velocity input; Height output
function [ Relative,Height] = ECEFVelocityToRelative(GPS,Velocity)
Relative = zeros(2,1);
GPS = reshape(GPS,1,[]);
GPS = GPS / norm(GPS);
% 求方向向量
East = cross(GPS,[0 1 0]);
North = cross(East,GPS);
Relative(1) = dot(North,Velocity);
Relative(2) = dot(East,Velocity);
Height = dot(GPS,Velocity);

== matlab function main/ECEFVelocityToRelative1 ==
  data: GPS input; Relative output; Velocity input; Height output
function [Relative,Height] = ECEFVelocityToRelative(GPS,Velocity)
Relative = zeros(2,1);
GPS = reshape(GPS,1,[]);
GPS = GPS / norm(GPS);
% 求方向向量
East = cross(GPS,[0 1 0]);
North = cross(East,GPS);
Relative(1) = dot(North,Velocity);
Relative(2) = dot(East,Velocity);
Height = dot(GPS,Velocity);

== stateflow chart main/Chart ==
  state Ascend
    DirectionEN = 0;
    Throttle = 1;
    TGTHeight = 250;
    End = 0;
    LowSinkRate = 0;
  state Go
    DirectionEN = 1;
    Throttle = 1;
    TGTHeight = 250;
    End = 0;
    LowSinkRate = 0;
  state Descend
    DirectionEN = 1;
    Throttle = 1;
    TGTHeight = HeightLand+10;
    End = 0;
    LowSinkRate = 0;
  state Landing
    DirectionEN = 1;
    Throttle = 1;
    TGTHeight = HeightLand-1;
    LowSinkRate = 1;
    End = 0;
  state Shutdown
    DirectionEN = 1;
    Throttle = 0;
    TGTHeight = HeightLand+0;
    End = 1;
    LowSinkRate = 0;
  (default) -> Ascend
  Ascend -> Go : [abs(Baro-TGTHeight) <10 && abs(VSpeed) < 1]
  Go -> Descend : [Distance < 10 && abs(HSpeed) <1]
  Descend -> Landing : [abs(Baro-TGTHeight) <10 && abs(VSpeed) < 1]
  Landing -> Shutdown : [abs(Baro-TGTHeight)  <5 && abs(VSpeed) < 1]
  data: DirectionEN output double; TGTHeight output double; Throttle output double; Baro input double; HeightLand input double; Distance input double; HSpeed input double; VSpeed input double; End output double =0; LowSinkRate output double
